simulink model "My_FilteredX_LMS_ANC"  (R2019b)
settings: Solver=FixedStepDiscrete  StartTime=0.0  StopTime=10  RelTol=1e-3
libraries: dspsnks4 x1, dspadpt3 x1, dspsrcs4 x1, dspvision x1
settings Model: SimulationMode=accelerator  Creator=The MathWorks, Inc.  LastModifiedBy=Administrator
settings DataIOCC: ReturnWorkspaceOutputs=off
settings DebuggingCC: ArithmeticOperatorsInVariantConditions=warning
settings SFSimCC: CustomCodeUndefinedFunction=UseInterfaceOnly

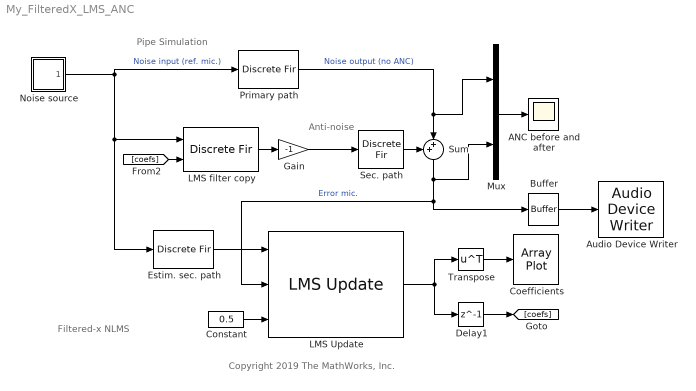
== system My_FilteredX_LMS_ANC ==
  note: Pipe Simulation
  note: Filtered-x NLMS
  note: Anti-noise
  note: Copyright 2019 The MathWorks, Inc.
  ANC before and after : Scope
  Audio Device Writer : dspsnks4/Audio Device Writer  Driver=DirectSound  Device=Default  InheritSampleRate=on  SampleRate=8000  BitDepth=16-bit integer  BufferSize=4096  NumBuffers=10  DefaultOutputChannelMapping=on  OutputChannelMapping=1:2  OutputNumUnderrunSamples=off  DriverIdx=1  DeviceWarnFlag=''
  Buffer : Buffer  N=4096  OutputFrames=off
  Coefficients : ArrayPlot
  Constant : Constant  Value=0.5
  Delay1 : Delay  DelayLength=1
  Estim. sec. path : DiscreteFir  Coefficients="[0.466  0.533  -0.257  -0.274  -0.231  -0.175]"
  Gain : Gain  Gain=-1
  LMS Update : dspadpt3/LMS Update  Method=Normalized LMS  Length=24  StepSizeSource=Input port  StepSize=0.1  LeakageFactor=1.0  InitialConditions=0  EnableAdaptInput=off  EnableResetInput=off  SimulateUsing=Interpreted execution
      settings: SourceProductName=DSP System Toolbox  SourceProductBaseCode=DS
  LMS filter copy : DiscreteFir  CoefSource=Input port
      settings: InputPortMap=u0,u1
  Mux : Mux  Inputs=2
  Noise source : Subsystem
  Primary path : DiscreteFir  Coefficients=conv([0.5 0.5 -.3 -.3 -.2 -.2],[.1 -.1 .2 -.2 .3 -.3 .15 -.15])
  Sec. path : DiscreteFir  Coefficients=[0.5 0.5 -.3 -.3 -.2 -.2]
  Sum : Sum  Inputs=++|
  Transpose : Math  Operator=transpose  SaturateOnIntegerOverflow=on
  wires:
  Primary path/1 -> Mux/1, Sum/2  "Noise output (no ANC)"
  LMS filter copy/1 -> Gain/1
  Sum/1 -> Buffer/1, LMS Update/2, Mux/2  "Error mic."
  Sec. path/1 -> Sum/1
  Estim. sec. path/1 -> LMS Update/1
  Mux/1 -> ANC before and after/1
  LMS Update/1 -> Transpose/1, Delay1/1
  [coefs] -> LMS filter copy/2
  Noise source/1(Synthesized Noise) -> Estim. sec. path/1, LMS filter copy/1, Primary path/1  "Noise input (ref. mic.)"
  Constant/1 -> LMS Update/3
  Transpose/1 -> Coefficients/1
  Delay1/1 -> [coefs]
  Gain/1 -> Sec. path/1
  Buffer/1 -> Audio Device Writer/1

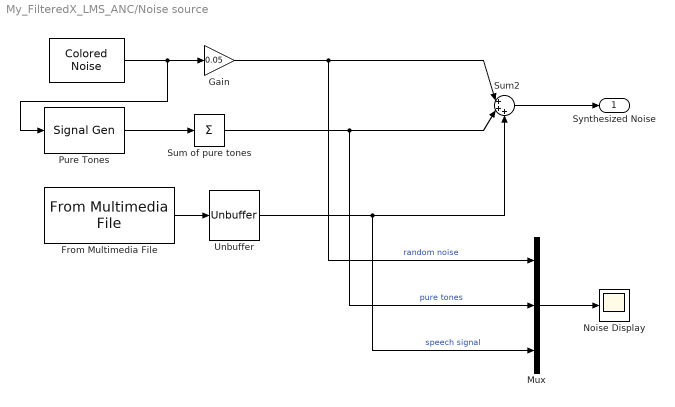
== system My_FilteredX_LMS_ANC/Noise source ==
  " " : dspsrcs4/Colored Noise  Color=white  InverseFrequencyPower=1  BoundedOutput=off  NumChannels=1  OutputDataType=double  SamplesPerFrame=1  SampleTime=1/8820  RandomStream=mt19937ar with seed  Seed=67  SimulateUsing=Interpreted execution
      settings: SourceProductName=DSP System Toolbox  SourceProductBaseCode=DS
  From Multimedia File : dspvision/From Multimedia File  inputFilename=.\speech3.wav  readRange=[1 Inf]  loop=on  numPlays=inf  outputStreams=Audio only  videoDataType=single  audioDataType=double  inheritSampleTime=on  userDefinedSampleTime=1/8820  noAudioOutput=off  isIntensityVideo=off  fourcc=RGB  colorVideoFormat=Separate color signals  outputEOF=off  dataOrg=Column-major  audioFrameSize=2048  computeAudioFrameSize=off  outSamplingMode=Sample based
      settings: SourceProductName=DSP System Toolbox  SourceProductBaseCode=DS
  Gain : Gain  Gain=0.05
  Mux : Mux  Inputs=3
  Noise Display : Scope
  Pure Tones : SignalGenerator  TimeSource=Use external signal  Amplitude=0.03  Frequency=[30 2000]
  Sum of pure tones : Sum  Inputs=+
  Sum2 : Sum  Inputs=|+++
  Unbuffer : Unbuffer
  Synthesized Noise : Outport  VectorParamsAs1DForOutWhenUnconnected=off
  wires:
  From Multimedia File/1 -> Unbuffer/1
  Gain/1 -> Mux/1, Sum2/1  "random noise"
  Mux/1 -> Noise Display/1
  Sum of pure tones/1 -> Mux/2, Sum2/2  "pure tones"
  Sum2/1 -> Synthesized Noise/1
  " "/1 -> Pure Tones/1, Gain/1
  Pure Tones/1 -> Sum of pure tones/1
  Unbuffer/1 -> Mux/3, Sum2/3  "speech signal"
